simulink model "Control_Scheme_Cartesian_PID_Simulink"  (R2021a)
settings: Solver=VariableStepAuto  StartTime=0.0  StopTime=8  RelTol=1e-20
libraries: simulink x10, pid_lib x6
(part 1 of 2)
settings Model: Creator=WU  LastModifiedBy=WU

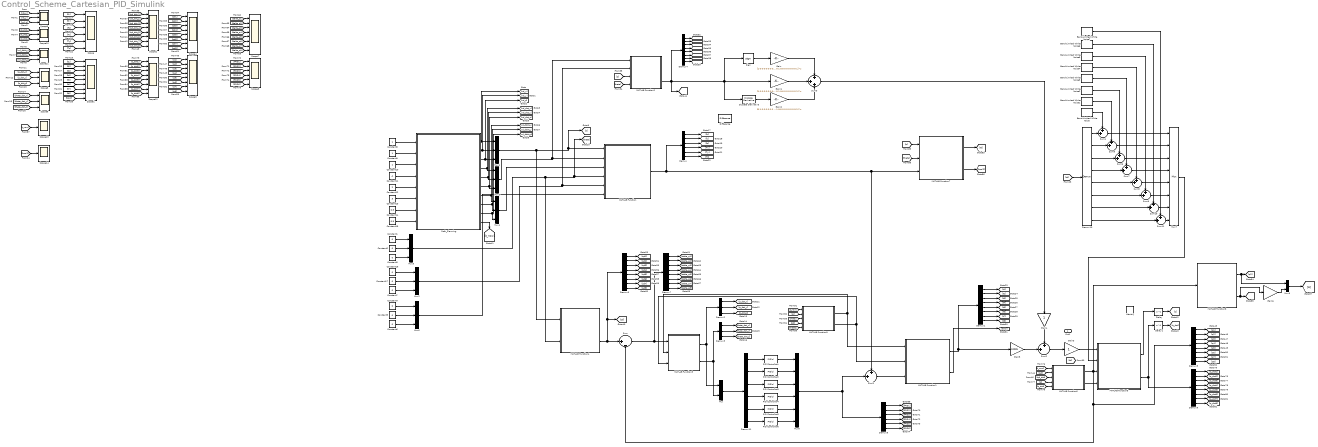
== system Control_Scheme_Cartesian_PID_Simulink ==
  Band-Limited White Noise : simulink/Sources/Band-Limited White Noise  Cov=[50]  Ts=0.001  seed=[23348]
  Band-Limited White Noise1 : simulink/Sources/Band-Limited White Noise  Cov=[50]  Ts=0.001  seed=[23347]
  Band-Limited White Noise2 : simulink/Sources/Band-Limited White Noise  Cov=[50]  Ts=0.001  seed=[23346]
  Band-Limited White Noise3 : simulink/Sources/Band-Limited White Noise  Cov=[50]  Ts=0.001  seed=[23345]
  Band-Limited White Noise4 : simulink/Sources/Band-Limited White Noise  Cov=[50]  Ts=0.001  seed=[23344]
  Band-Limited White Noise5 : simulink/Sources/Band-Limited White Noise  Cov=[50]  Ts=0.001  seed=[23343]
  Band-Limited White Noise6 : simulink/Sources/Band-Limited White Noise  Cov=[50]  Ts=0.001  seed=[23342]
  Band-Limited White Noise7 : simulink/Sources/Band-Limited White Noise  Cov=[50]  Ts=0.001  seed=[23341]
  Constant1 : Constant  Value=0  VectorParams1D=off
  Constant10 : Constant
  Constant11 : Constant  Value=-1
  Constant12 : Constant  Value=2
  Constant13 : Constant  Value=3
  Constant14 : Constant  Value=0.5
  Constant15 : Constant  Value=0.5
  Constant16 : Constant  Value=0  VectorParams1D=off
  Constant{2..3,5..7,17} (6 alike) : Constant  Value=0
  Constant4 : Constant  Value=0  VectorParams1D=off
  Constant8 : Constant  VectorParams1D=off
  Constant9 : Constant
  Delay : Delay  DelayLength=1
  Delay1 : Delay  DelayLength=1
  Demux : Demux  Outputs=6
      settings: DisplayOption=none
  Demux{1,4..7,9..10} (7 alike) : Demux  Outputs=8
      Demux1 settings: DisplayOption=none
      Demux10 settings: DisplayOption=none
      Demux4 settings: DisplayOption=none
  Demux11 : Demux  Outputs=6
      settings: DisplayOption=none
  Demux2 : Demux  Outputs=3
      settings: DisplayOption=none
  Demux3 : Demux  Outputs=3
      settings: DisplayOption=none
  Demux8 : Demux  Outputs=6
      settings: DisplayOption=none
  Difference : simulink/Discrete/Difference  ICPrevInput=0.0  OutMin=[]  OutMax=[]  OutDataType=fixdt(1, 16)  OutScaling=2^-10  DoSatur=off
  Discrete Derivative : simulink/Discrete/Discrete Derivative  gainval=1.0  ICPrevScaledInput=0.0  OutMin=[]  OutMax=[]  OutDataType=fixdt(1, 16)  OutScaling=2^-10  DoSatur=off
  Gain : Gain  Gain=[1 0 0 0 0 0 0 0;0 1 0 0 0 0 0 0;0 0 1 0 0 0 0 0;0 0 0 1 0 0 0 0;0 0 0 0 1 0 0 0;0 0 0 0 0 1 0 0;0 0 0 0 0 0 1 0;0 0 0 0 0 0 0 1]  Multiplication=Matrix(K*u) (u vector)
  Gain1 : Gain  Gain=[1 0 0 0 0 0 0 0;0 1 0 0 0 0 0 0;0 0 1 0 0 0 0 0;0 0 0 1 0 0 0 0;0 0 0 0 1 0 0 0;0 0 0 0 0 1 0 0;0 0 0 0 0 0 1 0;0 0 0 0 0 0 0 1]  Multiplication=Matrix(K*u) (u vector)
  Gain2 : Gain  Gain=[0.1 0 0 0 0 0 0 0;0 0.1 0 0 0 0 0 0;0 0 0.1 0 0 0 0 0;0 0 0 0.1 0 0 0 0;0 0 0 0 0.1 0 0 0;0 0 0 0 0 0.1 0 0;0 0 0 0 0 0 0.1 0;0 0 0 0 0 0 0 0.1]  Multiplication=Matrix(K*u) (u vector)
  Gain3 : Gain
  Gain4 : Gain
  Gain5 : Gain  Gain=0.0225
  Gain6 : Gain  Gain=3.14/180
  MATLAB Function : MATLAB Function  TreatAsAtomicUnit=on
  MATLAB Function1 : MATLAB Function  TreatAsAtomicUnit=on
  MATLAB Function2 : MATLAB Function  TreatAsAtomicUnit=on
  MATLAB Function3 : MATLAB Function  TreatAsAtomicUnit=on
  MATLAB Function4 : MATLAB Function  TreatAsAtomicUnit=on
  MATLAB Function5 : MATLAB Function  TreatAsAtomicUnit=on
  MATLAB Function6 : MATLAB Function  TreatAsAtomicUnit=on
  MATLAB Function7 : MATLAB Function  TreatAsAtomicUnit=on
  MATLAB Function8 : MATLAB Function  TreatAsAtomicUnit=on
  MATLAB Function9 : MATLAB Function  TreatAsAtomicUnit=on
  Memory : Memory
  Mux : Mux  Inputs=2
  Mux{1..6} (6 alike) : Mux  Inputs=3
  Mux7 : Mux  Inputs=8
  Mux8 : Mux  Inputs=6
  Mux9 : Mux  Inputs=2
  PID Controller{1..6} (6 alike) : pid_lib/PID Controller  Controller=PID  Form=Parallel  TimeDomain=Discrete-time  UseExternalTs=off  SampleTime=-1  IntegratorMethod=Forward Euler  FilterMethod=Forward Euler  ControllerParametersSource=internal  P=-150000  I=-1000  D=-100  UseFilter=on  N=100  TunerSelectOption=Transfer Function Based (PID Tuner App)  InitialConditionSource=internal  InitialConditionForIntegrator=0  InitialConditionForFilter=0  DifferentiatorICPrevScaledInput=0  ExternalReset=none  TrackingMode=off  Kt=1  LimitOutput=off  SatLimitsSource=internal  UpperSaturationLimit=inf  LowerSaturationLimit=-inf  LinearizeAsGain=on  AntiWindupMode=none  Kb=1  POutMin=[]  POutMax=[]  IOutMin=[]  IOutMax=[]  DOutMin=[]  DOutMax=[]  NOutMin=[]  NOutMax=[]  SumOutMin=[]  SumOutMax=[]  SaturationOutMin=[]  SaturationOutMax=[]  PParamMin=[]  PParamMax=[]  IParamMin=[]  IParamMax=[]  DParamMin=[]  DParamMax=[]  NParamMin=[]  NParamMax=[]  KbParamMin=[]  KbParamMax=[]  KtParamMin=[]  KtParamMax=[]  KbOutMin=[]  KbOutMax=[]  KtOutMin=[]  KtOutMax=[]  IntegratorOutMin=[]  IntegratorOutMax=[]  FilterOutMin=[]  FilterOutMax=[]  SumI1OutMin=[]  SumI1OutMax=[]  SumI2OutMin=[]  SumI2OutMax=[]  SumI3OutMin=[]  SumI3OutMax=[]  SumI4OutMin=[]  SumI4OutMax=[]  SumDOutMin=[]  SumDOutMax=[]  DifferentiatorOutMin=[]  DifferentiatorOutMax=[]  FilterDiffOutCoefMin=[]  FilterDiffOutCoefMax=[]  ReciprocalOutMin=[]  ReciprocalOutMax=[]  SumDenOutMin=[]  SumDenOutMax=[]  SumNumOutMin=[]  SumNumOutMax=[]  DivideOutMin=[]  DivideOutMax=[]  UdiffTsProdOutMin=[]  UdiffTsProdOutMax=[]  NTsProdOutMin=[]  NTsProdOutMax=[]  UintegralTsProdOutMin=[]  UintegralTsProdOutMax=[]  UngainTsProdOutMin=[]  UngainTsProdOutMax=[]  IntegratorContinuousStateAttributes=''  IntegratorStateMustResolveToSignalObject=off  IntegratorRTWStateStorageClass=Auto  FilterContinuousStateAttributes=''  FilterStateMustResolveToSignalObject=off  FilterRTWStateStorageClass=Auto  ParallelPVariant=InternalParameters  IdealPVariant=Disabled  IVariant=InternalParameters  DVariant=InternalParameters  IntegratorVariant=Discrete  SatVariant=Disabled  AWVariant=Passthrough  PCopyVariant=Disabled  TRVariant=Disabled  FdbkBlocksVariant=Forward  IdealPFdbkVariant=Disabled  SatFdbkVariant=Disabled  DerivativeFilterVariant=ForwardEulerFilter  NVariant=InternalParameters  NCopyVariant=Disabled  FilterICVariant=InternalICsFilter  IntegratorICVariant=InternalICs  ExternalResetVariant=Disabled  TRSumVariant=Passthrough  SumFdbkVariant=Disabled  SumVariant=Sum_PID  TsampFilterVariant=InternalTs  TsampNgainVariant=Passthrough  TsampIntegralVariant=Passthrough  ExternalSaturationOutDataTypeStr=Inherit: Same as second input
  Path_Planning : Subsystem
  Scope : Scope  NumInputPorts=6
  Scope1 : Scope  NumInputPorts=9
  Scope{5..6,9..11} (5 alike) : Scope  NumInputPorts=3
  Scope{2..4,7,12} (5 alike) : Scope  NumInputPorts=8
  Scope13 : Scope
  Scope14 : Scope
  Scope8 : Scope  NumInputPorts=6
  Sign : Signum
  Sum : Sum  Inputs=|+-
  Sum{1..2,4..11} (10 alike) : Sum  Inputs=++|
  Sum3 : Sum  Inputs=+++
  Out1 : Outport
  wires:
  Constant8/1 -> Path_Planning/1(xinit_x)  "xinit_x"
  Constant9/1 -> Path_Planning/2(xinit_y)  "xinit_y"
  Constant10/1 -> Path_Planning/3(xinit_z)  "xinit_z"
  Constant11/1 -> Path_Planning/4(xend_x)  "xend_x"
  Constant12/1 -> Path_Planning/5(xend_y)  "xend_y"
  Constant13/1 -> Path_Planning/6(xend_z)  "xend_z"
  Constant14/1 -> Path_Planning/7(vm)  "vm"
  Constant15/1 -> Path_Planning/8(am)  "am"
  Constant7/1 -> Mux2/3  "theta_dot_z"
  Constant17/1 -> Mux2/2  "theta_dot_y"
  Constant16/1 -> Mux2/1  "theta_dot_x"
  MATLAB Function/1(f) -> MATLAB Function7/3(we), Sum1/1, Demux/1  "fFF"
  Demux/1 -> [fx]  "fx"
  Demux/3 -> [fz]  "fz"
  Demux/4 -> [Tx]  "Tx"
  Demux/5 -> [Ty]  "Ty"
  Demux/6 -> [Tz]  "Tz"
  Path_Planning/1(xd_x) -> [xd_x], Mux1/1
  Path_Planning/3(xd_z) -> [xd_z], Mux1/3
  Path_Planning/4(xd_dot_x) -> [xd_dot_x], Mux3/1
  Path_Planning/5(xd_dot_y) -> [xd_dot_y], Mux3/2
  Path_Planning/6(xd_dot_z) -> [xd_dot_z], Mux3/3
  Path_Planning/7(xd_ddot_x) -> [xd_ddot_x], Mux4/1
  Path_Planning/8(xd_ddot_y) -> [xd_ddot_y], Mux4/2
  Path_Planning/9(xd_ddot_z) -> [xd_ddot_z], Mux4/3
  Path_Planning/2(xd_y) -> [xd_y], Mux1/2
  Constant1/1 -> Mux5/1  "theta_x"
  Constant2/1 -> Mux5/2  "theta_y"
  Constant3/1 -> Mux5/3  "theta_z"
  Mux5/1 -> MATLAB Function4/2(theta), [theta], MATLAB Function/4(theta)  "theta"
  MATLAB Function1/1(t) -> Gain5/1, Demux1/1  "t"
  Demux1/1 -> [t1]  "t1"
  Demux1/2 -> [t2]  "t2"
  Demux1/3 -> [t3]  "t3"
  Demux1/4 -> [t4]  "t4"
  Demux1/5 -> [t5]  "t5"
  Demux1/6 -> [t6]  "t6"
  Demux1/7 -> [t7]  "t7"
  Demux1/8 -> [t8]  "t8"
  MATLAB Function1/2(bool) -> [bool]
  MATLAB Function3/1(p_dot) -> Mux/1, Demux2/1
  Demux2/1 -> [p_dot_x]
  Demux2/2 -> [p_dot_y]
  Demux2/3 -> [p_dot_z]
  Demux3/1 -> [theta_dot_x]
  Demux3/3 -> [theta_dot_z]
  Demux3/2 -> [theta_dot_y]
  MATLAB Function3/2(theta_dot) -> Demux3/1, Mux/2
  Mux1/1 -> [p], MATLAB Function/1(p), MATLAB Function4/1(p)  "p"
  Mux3/1 -> MATLAB Function/2(p_dot), MATLAB Function2/1(p_dot)  "p_dot"
  Mux4/1 -> MATLAB Function/3(p_ddot)  "p_ddot"
  Constant6/1 -> Mux6/3  "theta_ddot_z"
  Constant4/1 -> Mux6/1  "theta_ddot_x"
  Constant5/1 -> Mux6/2  "theta_ddot_y"
  Mux2/1 -> MATLAB Function2/2(theta_dot), MATLAB Function/5(theta_dot)  "theta_dot"
  Mux6/1 -> MATLAB Function/6(theta_ddot)  "theta_ddot"
  MATLAB Function4/2(q) -> Demux6/1, [qd], Sum/1  "qd"
  [xd_x] -> Scope9/1
  [xd_y] -> Scope9/2
  [xd_z] -> Scope9/3
  [xd_dot_x] -> Scope10/1
  [xd_dot_y] -> Scope10/2
  [xd_ddot_x] -> Scope11/1
  [xd_ddot_y] -> Scope11/2
  [xd_ddot_z] -> Scope11/3
  Sum/1 -> Demux7/1, MATLAB Function3/1(q_dot)  "delta_q"
  MATLAB Function9/1(p_out) -> MATLAB Function3/2(p), MATLAB Function1/1(p)
  [p_dot_x] -> Scope5/1
  [p_dot_y] -> Scope5/2
  [p_dot_z] -> Scope5/3
  [theta_dot_x] -> Scope6/1
  [theta_dot_y] -> Scope6/2
  [theta_dot_z] -> Scope6/3
  Demux/2 -> [fy]  "fy"
  [fx] -> Scope/1
  [fy] -> Scope/2
  [fz] -> Scope/3
  [Tx] -> Scope/4
  [Ty] -> Scope/5
  [Tz] -> Scope/6
  MATLAB Function9/2(theta_out) -> MATLAB Function3/3(theta), MATLAB Function1/2(theta)
  [t1] -> Scope1/1
  [t4] -> Scope1/4
  [t8] -> Scope1/8
  [t5] -> Scope1/5
  [bool] -> Scope1/9
  [t7] -> Scope1/7
  [t6] -> Scope1/6
  [t3] -> Scope1/3
  [t2] -> Scope1/2
  [xd_dot_z] -> Scope10/3
  [p] -> MATLAB Function2/3(p)
  [theta] -> MATLAB Function2/4(theta)
  MATLAB Function2/2(q_dot) -> [qd_dot], Discrete Derivative/1, Gain1/1, Sign/1, Demux4/1  "q_dot"
  Demux4/1 -> [qd_dot_1]
  Demux4/2 -> [qd_dot_2]
  Demux4/3 -> [qd_dot_3]
  Demux4/4 -> [qd_dot_4]
  Demux4/5 -> [qd_dot_5]
  Demux4/6 -> [qd_dot_6]
  Demux4/7 -> [qd_dot_7]
  Demux4/8 -> [qd_dot_8]
  [qd_dot_1] -> Scope2/1
  [qd_dot_2] -> Scope2/2
  [qd_dot_4] -> Scope2/4
  [qd_dot_5] -> Scope2/5
  [qd_dot_6] -> Scope2/6
  [qd_dot_7] -> Scope2/7
  [qd_dot_8] -> Scope2/8
  [qd_dot_3] -> Scope2/3
  Discrete Derivative/1 -> Gain2/1
  Sign/1 -> Gain/1
  Gain1/1 -> Sum3/2
  Gain/1 -> Sum3/1
  Gain2/1 -> Sum3/3
  Gain3/1 -> MATLAB Function5/1(tao_in)  "tao_in"
  MATLAB Function5/1(q) -> Delay/1  "q"
  Path_Planning/10(t_now) -> [t_now]
  Demux5/1 -> [q1]
  Demux5/2 -> [q2]
  Demux5/3 -> [q3]
  Demux5/4 -> [q4]
  Demux5/7 -> [q7]
  Demux5/6 -> [q6]
  Demux5/8 -> [q8]
  Demux5/5 -> [q5]
  Demux6/3 -> [qd3]
  Demux6/4 -> [qd4]
  Demux6/7 -> [qd7]
  Demux6/1 -> [qd1]
  Demux6/5 -> [qd5]
  Demux6/6 -> [qd6]
  Demux6/8 -> [qd8]
  Demux6/2 -> [qd2]
  [q5] -> Scope3/5
  [q4] -> Scope3/4
  [q7] -> Scope3/7
  [q8] -> Scope3/8
  [q6] -> Scope3/6
  [q1] -> Scope3/1
  [q3] -> Scope3/3
  [q2] -> Scope3/2
  [qd8] -> Scope4/8
  [qd7] -> Scope4/7
  [qd5] -> Scope4/5
  [qd6] -> Scope4/6
  [qd2] -> Scope4/2
  [qd4] -> Scope4/4
  [qd3] -> Scope4/3
  [qd1] -> Scope4/1
  Demux7/8 -> [delta_q8]
  Demux7/2 -> [delta_q2]
  Demux7/3 -> [delta_q3]
  Demux7/7 -> [delta_q7]
  Demux7/4 -> [delta_q4]
  Demux7/5 -> [delta_q5]
  Demux7/1 -> [delta_q1]
  Demux7/6 -> [delta_q6]
  [delta_q1] -> Scope7/1
  [delta_q8] -> Scope7/8
  [delta_q3] -> Scope7/3
  [delta_q4] -> Scope7/4
  [delta_q5] -> Scope7/5
  [delta_q7] -> Scope7/7
  [delta_q6] -> Scope7/6
  [delta_q2] -> Scope7/2
  Demux8/4 -> [fPID4]  "fPID4"
  Demux8/5 -> [fPID5]  "fPID5"
  Demux8/1 -> [fPID1]  "fPID1"
  Demux8/2 -> [fPID2]  "fPID2"
  Demux8/3 -> [fPID3]  "fPID3"
  Demux8/6 -> [fPID6]  "fPID6"
  [fPID4] -> Scope8/4
  [fPID3] -> Scope8/3
  [fPID1] -> Scope8/1
  [fPID6] -> Scope8/6
  [fPID2] -> Scope8/2
  [fPID5] -> Scope8/5
  [qd] -> MATLAB Function6/2(qd)
  [t_now] -> MATLAB Function6/1(t)
  [qd_dot] -> MATLAB Function6/3(qd_dot)
  [q] -> MATLAB Function6/4(q)
  [q_dot] -> MATLAB Function6/5(q_dot)
  MATLAB Function6/1(q_1) -> Demux5/1, Sum/2, MATLAB Function8/1(q), MATLAB Function5/3(q_1)  "q"
  Delay/1 -> [q]
  MATLAB Function5/2(q_dot) -> Delay1/1, Demux9/1  "q_dot"
  Demux9/3 -> [q_dot3]
  Demux9/2 -> [q_dot2]
  Demux9/1 -> [q_dot1]
  Demux9/7 -> [q_dot7]
  Demux9/5 -> [q_dot5]
  Demux9/4 -> [q_dot4]
  Demux9/8 -> [q_dot8]
  Demux9/6 -> [q_dot6]
  [q_dot2] -> Scope12/2
  [q_dot8] -> Scope12/8
  [q_dot6] -> Scope12/6
  [q_dot7] -> Scope12/7
  [q_dot5] -> Scope12/5
  [q_dot3] -> Scope12/3
  [q_dot1] -> Scope12/1
  [q_dot4] -> Scope12/4
  [t_now] -> Scope13/1
  [theta] -> MATLAB Function7/2(theta)
  [p] -> MATLAB Function7/1(p)
  MATLAB Function7/1(t) -> [td]  "tTD"
  Sum2/1 -> Gain3/1
  Gain5/1 -> Sum2/2  "tao"
  MATLAB Function6/2(q_dot_1) -> MATLAB Function5/4(q_dot_1)  "q_dot_1"
  MATLAB Function8/1(p) -> Mux9/1, [p2]
  MATLAB Function8/2(theta) -> Gain6/1, [theta2]
  [p2] -> MATLAB Function9/4(p2)
  [t_now] -> MATLAB Function9/1(t_now)
  [theta2] -> MATLAB Function9/5(theta2)
  [theta] -> MATLAB Function9/3(theta)
  [p] -> MATLAB Function9/2(p)
  Gain4/1 -> Sum2/1  "taoff"
  Sum3/1 -> Gain4/1  "tFF"
  MATLAB Function7/2(bool) -> [bool2]
  [td] -> Demux10/1
  Demux10/1 -> Sum4/2
  Band-Limited White Noise/1 -> Sum4/1
  Sum4/1 -> Mux7/1
  Demux10/2 -> Sum5/2
  Sum5/1 -> Mux7/2
  Demux10/3 -> Sum6/2
  Sum6/1 -> Mux7/3
  Demux10/4 -> Sum7/2
  Sum7/1 -> Mux7/4
  Demux10/5 -> Sum8/2
  Sum8/1 -> Mux7/5
  Demux10/6 -> Sum9/2
  Sum9/1 -> Mux7/6
  Demux10/7 -> Sum10/2
  Sum10/1 -> Mux7/7
  Demux10/8 -> Sum11/2
  Sum11/1 -> Mux7/8
  Band-Limited White Noise1/1 -> Sum5/1
  Band-Limited White Noise2/1 -> Sum6/1
  Band-Limited White Noise3/1 -> Sum7/1
  Band-Limited White Noise4/1 -> Sum8/1
  Band-Limited White Noise5/1 -> Sum9/1
  Band-Limited White Noise6/1 -> Sum10/1
  Band-Limited White Noise7/1 -> Sum11/1
  Mux/1 -> Demux11/1  "delta_x"
  Demux11/1 -> PID Controller1/1
  Demux11/2 -> PID Controller2/1
  PID Controller1/1 -> Mux8/1  "fPID"
  PID Controller2/1 -> Mux8/2  "fPID"
  Demux11/4 -> PID Controller4/1
  PID Controller4/1 -> Mux8/4  "fPID"
  Demux11/3 -> PID Controller3/1
  PID Controller3/1 -> Mux8/3  "fPID"
  PID Controller5/1 -> Mux8/5  "fPID"
  PID Controller6/1 -> Mux8/6  "fPID"
  Demux11/6 -> PID Controller6/1
  Mux8/1 -> Sum1/2, Demux8/1  "fPID"
  [bool2] -> Scope14/1
  Delay1/1 -> [q_dot]
  Mux7/1 -> MATLAB Function5/2(t_in)
  Mux9/1 -> [A]  "x"
  Gain6/1 -> Mux9/2
  Demux11/5 -> PID Controller5/1
  Sum1/1 -> MATLAB Function1/3(we)  "f"

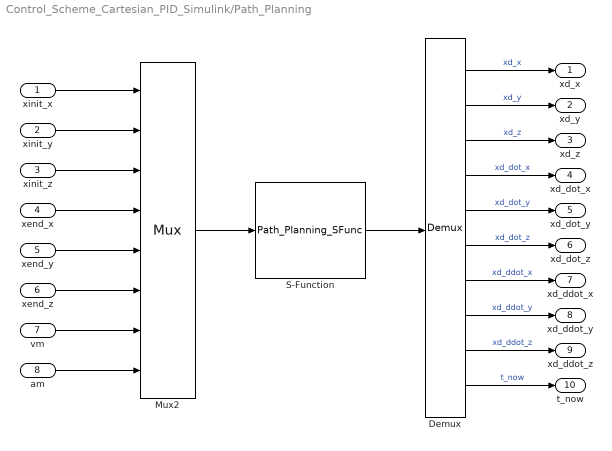
== system Control_Scheme_Cartesian_PID_Simulink/Path_Planning ==
  xinit_x : Inport
  xinit_y : Inport  Port=2
  xinit_z : Inport  Port=3
  xend_x : Inport  Port=4
  xend_y : Inport  Port=5
  xend_z : Inport  Port=6
  vm : Inport  Port=7
  am : Inport  Port=8
  Demux : Demux  Outputs=10
      settings: DisplayOption=none
  Mux2 : Mux  Inputs=8
  S-Function : S-Function  FunctionName=Path_Planning_SFunc  SFunctionDeploymentMode=off  EnableBusSupport=off
  xd_x : Outport
  xd_y : Outport  Port=2
  xd_z : Outport  Port=3
  xd_dot_x : Outport  Port=4
  xd_dot_y : Outport  Port=5
  xd_dot_z : Outport  Port=6
  xd_ddot_x : Outport  Port=7
  xd_ddot_y : Outport  Port=8
  xd_ddot_z : Outport  Port=9
  t_now : Outport  Port=10
  wires:
  Demux/7 -> xd_ddot_x/1  "xd_ddot_x"
  vm/1 -> Mux2/7
  xinit_y/1 -> Mux2/2
  Demux/1 -> xd_x/1  "xd_x"
  Demux/4 -> xd_dot_x/1  "xd_dot_x"
  Demux/5 -> xd_dot_y/1  "xd_dot_y"
  Demux/9 -> xd_ddot_z/1  "xd_ddot_z"
  Demux/8 -> xd_ddot_y/1  "xd_ddot_y"
  Demux/3 -> xd_z/1  "xd_z"
  Demux/6 -> xd_dot_z/1  "xd_dot_z"
  Demux/2 -> xd_y/1  "xd_y"
  xend_y/1 -> Mux2/5
  Mux2/1 -> S-Function/1
  S-Function/1 -> Demux/1
  xend_z/1 -> Mux2/6
  xend_x/1 -> Mux2/4
  xinit_z/1 -> Mux2/3
  xinit_x/1 -> Mux2/1
  am/1 -> Mux2/8
  Demux/10 -> t_now/1  "t_now"

== matlab function Control_Scheme_Cartesian_PID_Simulink/MATLAB Function9 ==
  data: t_now input; p_out output; p input; theta input; p2 input; theta2 input; theta_out output
function [p_out,theta_out]= Select_p_and_theta(t_now,p,theta,p2,theta2)
p_out=zeros(3,1);
theta_out=zeros(3,1);

if t_now<=1e-3
    p_out=p;
    theta_out=theta;
else
    p_out=p2;
    theta_out=theta2;
end
p_out=p;
theta_out=theta;


end

== matlab function Control_Scheme_Cartesian_PID_Simulink/MATLAB Function1 ==
  data: p input; t output; theta input; we input; bool output
function [t,bool] = Tension_Distribution_Func(p,theta,we)
% 求解索力分布的函数
% 输入：p 动平台位置 3*1
%      theta 动平台坐标系XYZ欧拉角 3*1
%      we 动平台受到的wrench 6*1(包含本身质量)
% 输出：t 绳索的张力的大小 8*1

g=9.81; %重力加速度
theta=theta';
x=theta(1);
y=theta(2);
z=theta(3);
Rxyz=Theta2RotationMatrix_Func(x,y,z);
f=we;
%% CoGiRo的参数 8绳索6自由度的CDPRs
% ai的定义
a1=[-7.5 -5.5 6]';
a2=[-7.5 -5.5 6]';
a3=[-7.5 5.5 6]';
a4=[-7.5 5.5 6]';
a5=[7.5 5.5 6]';
a6=[7.5 5.5 6]';
a7=[7.5 -5.5 6]';
a8=[7.5 -5.5 6]';
% bi的定义
b1=Rxyz*[0.5 -0.5 0]';
b2=Rxyz*[-0.5 0.5 1]';
b3=Rxyz*[-0.5 -0.5 0]';
b4=Rxyz*[0.5 0.5 1]';
b5=Rxyz*[-0.5 0.5 0]';
b6=Rxyz*[0.5 -0.5 1]';
b7=Rxyz*[0.5 0.5 0]';
b8=Rxyz*[-0.5 -0.5 1]';
% 绳索张力的上下限
tM=1000;
tm=10;
%% li=ai-bi-p,然后归一化li得到si=li/norm(li)
% li=ai-bi-p
l1=a1-b1-p;
l2=a2-b2-p;
l3=a3-b3-p;
l4=a4-b4-p;
l5=a5-b5-p;
l6=a6-b6-p;
l7=a7-b7-p;
l8=a8-b8-p;
% for i=1:8
%     expr=['l',num2str(i),'=a',num2str(i),'-b',num2str(i),'-p;'];
%     eval(expr);
% end
% si=li/norm(li)
s1=l1/norm(l1);
s2=l2/norm(l2);
s3=l3/norm(l3);
s4=l4/norm(l4);
s5=l5/norm(l5);
s6=l6/norm(l6);
s7=l7/norm(l7);
s8=l8/norm(l8);

% for i=1:8
%     expr=['s',num2str(i),'=l',num2str(i),'./norm(l',num2str(i),');'];
%     eval(expr);
% end

%% 构建W矩阵
% wi=[si;cross(bi,si)]
w1=[s1;cross(b1,s1)];
w2=[s2;cross(b2,s2)];
w3=[s3;cross(b3,s3)];
w4=[s4;cross(b4,s4)];
w5=[s5;cross(b5,s5)];
w6=[s6;cross(b6,s6)];
w7=[s7;cross(b7,s7)];
w8=[s8;cross(b8,s8)];
W=[w1 w2 w3 w4 w5 w6 w7 w8];

W_plus=pinv(W);
N=null(W);
tp=W_plus*f;

tm_vec=[tm;tm;tm;tm;tm;tm;tm;tm;];
tM_vec=[tM;tM;tM;tM;tM;tM;tM;tM;];

% line_select=[];
% langda_select=[];

find=0;
k_vector_all=[1;2;3;4;5;6;7;8];

%% 寻找第一个顶点vinit
i=1;
j=2;
bi=tm;
bj=tm;
bk_1=0;
bk_2=0;
ni=N(i,:);
nj=N(j,:);
tpi=tp(i,:);
tpj=tp(j,:);
A=[ni;nj];
b=[bi-tpi;bj-tpj];
langda=A\b; %2*1向量
vij=langda;

% line_select=[line_select;j];
% line_select=[line_select;i];
line_select=[i];

lk_1=i;
lk_2=j;

% line_find=[];
% line_find=[line_find;1];
% line_find=[line_find;2];
line_find=[i;j];

for i=3:8
    ni_2=N(i,:);
    tpi_2=tp(i,:);
    if ni_2*langda>=tm-tpi_2 & ni_2*langda<=tM-tpi_2
        line_find=[line_find;i];
    end
    
end

langda_select=[vij];


k_vector=setdiff(k_vector_all,line_select);

%% 循环找下一个节点，直到找到vk==vf
vk=[1e30;1e30];
% alpah_v=[1e30;1e30];
alpah_v=[1e30];
vk_1=vij;
nk_1=ni;
nk_2=nj;
nk_1_vertical=null(nk_1)';
nk_2_vertical=null(nk_2)';
l=0;
bk=0;
tpk=0;
count=0;
find2=0;
vf=vij;
vf_count=count+1;
nk_1_vertical_final=[0 0];
while(1)
%     alpah_k=[1e30;1e30];
    alpah_k=[1e30];
    count=count+1;
    find2=0;
    nk_1_vertical_final=[0 0];
    for i=1:length(k_vector)
        k=k_vector(i);
        nk=N(k,:);
        tpk=tp(k,:);
        
        % 考虑bj=tm情况
        if bk_2==0           
            nk_1_vertical_1=[nk_1(2) -nk_1(1)];
            nk_1_vertical_2=[-nk_1(2) nk_1(1)];
%             nk_1_vertical_1=[-nk_1(2) nk_1(1)];
%             nk_1_vertical_2=[nk_1(2) -nk_1(1)];
            if nk_2*nk_1_vertical_1'>=0
                nk_1_vertical=nk_1_vertical_1;
            else
                nk_1_vertical=nk_1_vertical_2;
            end           
            
            if nk*nk_1_vertical'>0
                if k==lk_2
                    if nk*vk_1<=tm-tpk
                        alpah_k=(tM-tpk-nk*vk_1)/(nk*nk_1_vertical');
                        bk_tmp=1;
                    elseif nk*vk_1>tm-tpk & nk*vk_1<=tM-tpk
                        alpah_k=(tM-tpk-nk*vk_1)/(nk*nk_1_vertical');
                        bk_tmp=1;
                    else
                        bk_tmp=0;
                    end
%                     if nk*vk_1>tm-tpk & nk*vk_1<=tM-tpk
%                         alpah_k=(tM-tpk-nk*vk_1)/(nk*nk_1_vertical');
%                         bk_tmp=1;
%                     end
                else
                    if nk*vk_1<=tm-tpk
                        alpah_k=(tm-tpk-nk*vk_1)/(nk*nk_1_vertical');
                        bk_tmp=0;
                    elseif nk*vk_1>tm-tpk & nk*vk_1<=tM-tpk
                        alpah_k=(tM-tpk-nk*vk_1)/(nk*nk_1_vertical');
                        bk_tmp=1;
                    else
                        bk_tmp=0;
                    end
%                     if nk*vk_1>tm-tpk & nk*vk_1<=tM-tpk
%                         alpah_k=(tM-tpk-nk*vk_1)/(nk*nk_1_vertical');
%                         bk_tmp=1;
%                     end
                end
                if (alpah_k<alpah_v) & alpah_k>=1e-6
                    alpah_v=alpah_k;
                    l=k;
                    find2=1;
                    nk_1_vertical_final=nk_1_vertical;
                    bk=bk_tmp;
                else
                    
                end
            end

            if nk*nk_1_vertical'<0
                if k==lk_2
                    if nk*vk_1>=tM-tpk
                        alpah_k=(tm-tpk-nk*vk_1)/(nk*nk_1_vertical');
                        bk_tmp=0;
                    elseif nk*vk_1>=tm-tpk & nk*vk_1<tM-tpk
                        alpah_k=(tm-tpk-nk*vk_1)/(nk*nk_1_vertical');
                        bk_tmp=0;
                    else
                        bk_tmp=0;
                    end
%                     if nk*vk_1>=tm-tpk & nk*vk_1<tM-tpk
%                         alpah_k=(tm-tpk-nk*vk_1)/(nk*nk_1_vertical');
%                         bk_tmp=0;
%                     end
                else
                    if nk*vk_1>=tM-tpk
                        alpah_k=(tM-tpk-nk*vk_1)/(nk*nk_1_vertical');
                        bk_tmp=1;
                    elseif nk*vk_1>=tm-tpk & nk*vk_1<tM-tpk
                        alpah_k=(tm-tpk-nk*vk_1)/(nk*nk_1_vertical');
                        bk_tmp=0;
                    else
                        bk_tmp=0;
                    end
%                     if nk*vk_1>=tm-tpk & nk*vk_1<tM-tpk
%                         alpah_k=(tm-tpk-nk*vk_1)/(nk*nk_1_vertical');
%                         bk_tmp=0;
%                     end
                end
                if (alpah_k<alpah_v) & alpah_k>=1e-6
                    alpah_v=alpah_k;
                    l=k;
                    find2=1;
                    nk_1_vertical_final=nk_1_vertical;
                    bk=bk_tmp;
                else
                    
                end
            end
        
        % 考虑bk=tM的情况
        elseif bk_2==1
            nk_1_vertical_1=[nk_1(2) -nk_1(1)];
            nk_1_vertical_2=[-nk_1(2) nk_1(1)];
%             nk_1_vertical_1=[-nk_1(2) nk_1(1)];
%             nk_1_vertical_2=[nk_1(2) -nk_1(1)];
            if nk_2*nk_1_vertical_1'<=0
                nk_1_vertical=nk_1_vertical_1;
            else
                nk_1_vertical=nk_1_vertical_2;
            end

            if nk*nk_1_vertical'>0
                if k==lk_2
                    if nk*vk_1<=tm-tpk
                        alpah_k=(tM-tpk-nk*vk_1)/(nk*nk_1_vertical');
                        bk_tmp=1;
                    elseif nk*vk_1>tm-tpk & nk*vk_1<=tM-tpk
                        alpah_k=(tM-tpk-nk*vk_1)/(nk*nk_1_vertical');
                        bk_tmp=1;
                    else
                        bk_tmp=0;
                    end
%                     if nk*vk_1>tm-tpk & nk*vk_1<=tM-tpk
%                         alpah_k=(tM-tpk-nk*vk_1)/(nk*nk_1_vertical');
%                         bk_tmp=1;
%                     end
                else
                    if nk*vk_1<=tm-tpk
                        alpah_k=(tm-tpk-nk*vk_1)/(nk*nk_1_vertical');
                        bk_tmp=0;
                    elseif nk*vk_1>tm-tpk & nk*vk_1<=tM-tpk
                        alpah_k=(tM-tpk-nk*vk_1)/(nk*nk_1_vertical');
                        bk_tmp=1;
                    else
                        bk_tmp=0;
                    end
%                     if nk*vk_1>tm-tpk & nk*vk_1<=tM-tpk
%                         alpah_k=(tM-tpk-nk*vk_1)/(nk*nk_1_vertical');
%                         bk_tmp=1;
%                     end
                end
                if (alpah_k<alpah_v) & alpah_k>=1e-6
                    alpah_v=alpah_k;
                    l=k;
                    find2=1;
                    nk_1_vertical_final=nk_1_vertical;
                    bk=bk_tmp;
                else
                    
                end
            end

            if nk*nk_1_vertical'<0
                if k==lk_2
                    if nk*vk_1>=tM-tpk
                        alpah_k=(tm-tpk-nk*vk_1)/(nk*nk_1_vertical');
                        bk_tmp=0;
                    elseif nk*vk_1>=tm-tpk & nk*vk_1<tM-tpk
                        alpah_k=(tm-tpk-nk*vk_1)/(nk*nk_1_vertical');
                        bk_tmp=0;
                    else
                        bk_tmp=0;
                    end
%                     if nk*vk_1>=tm-tpk & nk*vk_1<tM-tpk
%                         alpah_k=(tm-tpk-nk*vk_1)/(nk*nk_1_vertical');
%                         bk_tmp=0;
%                     end
                else
                    if nk*vk_1>=tM-tpk
                        alpah_k=(tM-tpk-nk*vk_1)/(nk*nk_1_vertical');
                        bk_tmp=1;
                    elseif nk*vk_1>=tm-tpk & nk*vk_1<tM-tpk
                        alpah_k=(tm-tpk-nk*vk_1)/(nk*nk_1_vertical');
                        bk_tmp=0;
                    else
                        bk_tmp=0;
                    end
%                     if nk*vk_1>=tm-tpk & nk*vk_1<tM-tpk
%                         alpah_k=(tm-tpk-nk*vk_1)/(nk*nk_1_vertical');
%                         bk_tmp=0;
%                     end
                end
                if (alpah_k<alpah_v) & alpah_k>=1e-6
                    alpah_v=alpah_k;
                    l=k;
                    find2=1;
                    nk_1_vertical_final=nk_1_vertical;
                    bk=bk_tmp;
                else
                    
                end
            end
        else
            find2=0;
        end
    end
    if find2==0 || count>1000
        t=[0 0 0 0 0 0 0 0]';
        bool=0;
%         disp("索力分布无解");
        break
    else
        vk=vk_1+alpah_v.*nk_1_vertical_final';
        nk=N(l,:);
        langda_select=[langda_select,vk];
    %     line_select(1,:)=line_select(2,:);
    %     line_select(2,:)=l;
        line_select(1)=l;
        lk=l;
        k_vector=setdiff(k_vector_all,line_select);
        vk_2=vk_1;
        vk_1=vk;
        nk_2=nk_1;
        nk_1=nk;
        bk_2=bk_1;
        bk_1=bk;
        lk_2=lk_1;
        lk_1=lk;
    %     alpah_v=[1e10;1e10];
        alpah_v=[1e30];

        if ~ismember(l,line_find)
            line_find=[line_find;l];
            line_find=sort(line_find);
            vf=vk;
            vf_count=count+1;
        else
            if abs(vf(1)-vk(1))<1e-3 & abs(vf(2)-vk(2))<1e-3
                line_find=sort(line_find);
                if isequal(line_find,k_vector_all)
%                     disp('查找成功');
                    bool=1;
                    break;
                else
                    t=[0 0 0 0 0 0 0 0]';
                    bool=0;
%                     disp('查找失败');
                    return
                end
            else
                line_find=line_find;
            end
        end        
    end
    
end

langda_final_vce=langda_select(1:2,end-(size(langda_select,2)-vf_count):end-1);

%% 重心法得到多边形质心
% 求解A
A=0;
vc1=0;
vc2=0;

count=size(langda_select,2)-vf_count;

if count==3
    vc1=(langda_final_vce(1,1)+langda_final_vce(1,2)+langda_final_vce(1,3))/3;
    vc2=(langda_final_vce(2,1)+langda_final_vce(2,2)+langda_final_vce(2,3))/3;
end

if count==4
    vc1=(langda_final_vce(1,1)+langda_final_vce(1,2)+langda_final_vce(1,3)+langda_final_vce(1,4))/4;
    vc2=(langda_final_vce(2,1)+langda_final_vce(2,2)+langda_final_vce(2,3)+langda_final_vce(2,4))/4;
end

if count>4
    for p=1:size(langda_final_vce,2)-1
        A=A+(langda_final_vce(1,p)*langda_final_vce(2,p+1)-langda_final_vce(1,p+1)*langda_final_vce(2,p))/2;
    end

    for p=1:size(langda_final_vce,2)-1
        vc1=vc1+((langda_final_vce(1,p)+langda_final_vce(1,p+1))*(langda_final_vce(1,p)*langda_final_vce(2,p+1)-langda_final_vce(1,p+1)*langda_final_vce(2,p)))/(6*A);
        vc2=vc2+((langda_final_vce(2,p)+langda_final_vce(2,p+1))*(langda_final_vce(1,p)*langda_final_vce(2,p+1)-langda_final_vce(1,p+1)*langda_final_vce(2,p)))/(6*A);
    end
end

% vc1=456.6389;
% vc2=534.3178;

t=zeros(8,1);

langda_final=[vc1 vc2]';
t=tp+N*langda_final;

end

== matlab function Control_Scheme_Cartesian_PID_Simulink/MATLAB Function ==
  data: p input; f output; p_dot input; p_ddot input; theta input; theta_dot input; theta_ddot input
function f  = Inverse_Dynamics_Func(p,p_dot,p_ddot,theta,theta_dot,theta_ddot)
% CDPRs的动力学求解
% 输入:p,p_dot,p_ddot,theta,theta_dot,theta_ddot 位置与姿态及其各阶导数
% 输出:f 动平台产生的wrench
mp=79;          %动平台质量
g=9.81;
cp=[0 -0.075 0]'; %动平台COM相对于动平台的原点的位置偏移
IG=[1 0 0;0 1 0;0 0 1]; %动平台相对于动平台坐标系的惯性矩阵

% x_dot=[p_dot;theta_dot];
% x_ddot=[p_ddot;theta_ddot];
x_dot=[p_dot;theta_dot];
x_ddot=[p_ddot;theta_ddot];

%% 得到旋转矩阵
Rxyz=Theta2RotationMatrix_Func(theta(1),theta(2),theta(3));

%% 得到S(x),在得到平台在世界坐标系下的角速度omiga,进而得到omiga^是omiga对应的斜对称矩阵
thetax=theta(1);
thetay=theta(2);
thetaz=theta(3);

thetax_dot=theta_dot(1);
thetay_dot=theta_dot(2);
thetaz_dot=theta_dot(3);

Sx=[1 0 sind(thetay); 0 cosd(thetax) -sind(thetax)*cosd(thetay); 0 sind(thetax) cosd(thetax)*cosd(thetay)];
omiga=Sx*theta_dot;
v1=omiga(1);
v2=omiga(2);
v3=omiga(3);
omiga_sharp=[0 -v3 v2;v3 0 -v1;-v2 v1 0];
Sx=[eye(3,3) zeros(3,3); zeros(3,3) Sx];

%% 得到S_dot_(x,x_dot)的每个元素为S(x)相应位置元素的导数
Sx_dot_2_2=[0 0 cosd(thetay)*thetay_dot;0 -sind(thetax)*thetax_dot -cosd(thetax)*cosd(thetay)*thetax_dot+sind(thetax)*sind(thetay)*thetay_dot; 0 cosd(thetax)*thetax_dot -sind(thetax)*cosd(thetay)*thetax_dot-cosd(thetax)*sind(thetay)*thetay_dot];
Sx_dot=[zeros(3,3) zeros(3,3);zeros(3,3) Sx_dot_2_2];
% Sx_dot=zeros(6,6); %简化使得导数均为0

%% 通过cp得到c(x)=Rxyz*cp,进而得到c^(x)是c(x)对应的斜对称矩阵
cx=Rxyz*cp;
v1=cx(1);
v2=cx(2);
v3=cx(3);
c_sharp_x=[0 -v3 v2;v3 0 -v1;-v2 v1 0];

%% 得到g(x)
gx=mp*g*[0 0 -1 -cx(2) cx(1) 0]';

%% 得到H(x)=Rxyz*IG*Rxyz'+mp*c_sharp_x*c_sharp_x';
Hx=Rxyz*IG*Rxyz'+mp*c_sharp_x*c_sharp_x';

%% 得到M'(x)
M_apo_x=[mp*ones(3,3) -mp*c_sharp_x; mp*c_sharp_x Hx];

%% 得到C'(x)
C_apo_x=[mp*omiga_sharp*omiga_sharp*cx; omiga_sharp*Hx*omiga];

%% 最终得到动平台上wrench f
f=(M_apo_x*(Sx_dot*x_dot+Sx*x_ddot)+C_apo_x-gx);
end

== matlab function Control_Scheme_Cartesian_PID_Simulink/MATLAB Function2 ==
  data: p_dot input; theta_dot input; l_dot output; p input; theta input; q_dot output
function [l_dot,q_dot] = Jacobian_Func(p_dot,theta_dot,p,theta)
% 雅可比矩阵，从位姿x到绳长l，再到电机角度q

x=theta(1);
y=theta(2);
z=theta(3);
Rxyz=Theta2RotationMatrix_Func(x,y,z);

%% CoGiRo的参数 8绳索6自由度的CDPRs
% ai的定义
a1=[-7.5 -5.5 6]';
a2=[-7.5 -5.5 6]';
a3=[-7.5 5.5 6]';
a4=[-7.5 5.5 6]';
a5=[7.5 5.5 6]';
a6=[7.5 5.5 6]';
a7=[7.5 -5.5 6]';
a8=[7.5 -5.5 6]';
% bi的定义
b1=Rxyz*[0.5 -0.5 0]';
b2=Rxyz*[-0.5 0.5 1]';
b3=Rxyz*[-0.5 -0.5 0]';
b4=Rxyz*[0.5 0.5 1]';
b5=Rxyz*[-0.5 0.5 0]';
b6=Rxyz*[0.5 -0.5 1]';
b7=Rxyz*[0.5 0.5 0]';
b8=Rxyz*[-0.5 -0.5 1]';
% 绳索张力的上下限
tM=1000;
tm=10;
%% li=ai-bi-p,然后归一化li得到si=li/norm(li)
% li=ai-bi-p
l1=a1-b1-p;
l2=a2-b2-p;
l3=a3-b3-p;
l4=a4-b4-p;
l5=a5-b5-p;
l6=a6-b6-p;
l7=a7-b7-p;
l8=a8-b8-p;
% for i=1:8
%     expr=['l',num2str(i),'=a',num2str(i),'-b',num2str(i),'-p;'];
%     eval(expr);
% end
% si=li/norm(li)
s1=l1/norm(l1);
s2=l2/norm(l2);
s3=l3/norm(l3);
s4=l4/norm(l4);
s5=l5/norm(l5);
s6=l6/norm(l6);
s7=l7/norm(l7);
s8=l8/norm(l8);
% for i=1:8
%     expr=['s',num2str(i),'=l',num2str(i),'./norm(l',num2str(i),');'];
%     eval(expr);
% end

%% 构建W矩阵
% wi=[si;cross(bi,si)]
w1=[s1;cross(b1,s1)];
w2=[s2;cross(b2,s2)];
w3=[s3;cross(b3,s3)];
w4=[s4;cross(b4,s4)];
w5=[s5;cross(b5,s5)];
w6=[s6;cross(b6,s6)];
w7=[s7;cross(b7,s7)];
w8=[s8;cross(b8,s8)];
W=[w1 w2 w3 w4 w5 w6 w7 w8];

%% 得到雅可比矩阵
J=-W';

x_dot=[p_dot;theta_dot];

l_dot=J*x_dot;
q_dot=l_dot/0.0225;

end

== matlab function Control_Scheme_Cartesian_PID_Simulink/MATLAB Function3 ==
  data: q_dot input; p_dot output; p input; theta input; theta_dot output
function [p_dot,theta_dot] = Inverse_Jacobian_Func(q_dot,p,theta)
% 雅可比矩阵，从位姿x到绳长l，再到电机角度q

x=theta(1);
y=theta(2);
z=theta(3);
Rxyz=Theta2RotationMatrix_Func(x,y,z);

%% CoGiRo的参数 8绳索6自由度的CDPRs
% ai的定义
a1=[-7.5 -5.5 6]';
a2=[-7.5 -5.5 6]';
a3=[-7.5 5.5 6]';
a4=[-7.5 5.5 6]';
a5=[7.5 5.5 6]';
a6=[7.5 5.5 6]';
a7=[7.5 -5.5 6]';
a8=[7.5 -5.5 6]';
% bi的定义
b1=Rxyz*[0.5 -0.5 0]';
b2=Rxyz*[-0.5 0.5 1]';
b3=Rxyz*[-0.5 -0.5 0]';
b4=Rxyz*[0.5 0.5 1]';
b5=Rxyz*[-0.5 0.5 0]';
b6=Rxyz*[0.5 -0.5 1]';
b7=Rxyz*[0.5 0.5 0]';
b8=Rxyz*[-0.5 -0.5 1]';
% 绳索张力的上下限
tM=1000;
tm=10;
%% li=ai-bi-p,然后归一化li得到si=li/norm(li)
% li=ai-bi-p
l1=a1-b1-p;
l2=a2-b2-p;
l3=a3-b3-p;
l4=a4-b4-p;
l5=a5-b5-p;
l6=a6-b6-p;
l7=a7-b7-p;
l8=a8-b8-p;
% for i=1:8
%     expr=['l',num2str(i),'=a',num2str(i),'-b',num2str(i),'-p;'];
%     eval(expr);
% end
% si=li/norm(li)
s1=l1/norm(l1);
s2=l2/norm(l2);
s3=l3/norm(l3);
s4=l4/norm(l4);
s5=l5/norm(l5);
s6=l6/norm(l6);
s7=l7/norm(l7);
s8=l8/norm(l8);
% for i=1:8
%     expr=['s',num2str(i),'=l',num2str(i),'./norm(l',num2str(i),');'];
%     eval(expr);
% end

%% 构建W矩阵
% wi=[si;cross(bi,si)]
w1=[s1;cross(b1,s1)];
w2=[s2;cross(b2,s2)];
w3=[s3;cross(b3,s3)];
w4=[s4;cross(b4,s4)];
w5=[s5;cross(b5,s5)];
w6=[s6;cross(b6,s6)];
w7=[s7;cross(b7,s7)];
w8=[s8;cross(b8,s8)];
W=[w1 w2 w3 w4 w5 w6 w7 w8];

%% 得到雅可比矩阵
J=-W';
J_plus=pinv(J);
l_dot=q_dot*0.0225;
x_dot=J_plus*l_dot;
p_dot=x_dot(1:3,:);
theta_dot=x_dot(4:6,:);
% if theta_dot(1)<1e-3
%     theta_dot(1)=0;
% end
% if theta_dot(2)<1e-3
%     theta_dot(2)=0;
% end
% if theta_dot(3)<1e-3
%     theta_dot(3)=0;
% end
end

== matlab function Control_Scheme_Cartesian_PID_Simulink/MATLAB Function4 ==
  data: p input; l_len output; theta input; q output
function [l_len,q]  = InverseKenematics_Func(p,theta)
%UNTITLED3 求解CDPRs的逆运动学解
%   Detailed explanation goes here
x=theta(1);
y=theta(2);
z=theta(3);
Rxyz=Theta2RotationMatrix_Func(x,y,z);
%% CoGiRo的参数 8绳索6自由度的CDPRs
% ai的定义
a1=[-7.5 -5.5 6]';
a2=[-7.5 -5.5 6]';
a3=[-7.5 5.5 6]';
a4=[-7.5 5.5 6]';
a5=[7.5 5.5 6]';
a6=[7.5 5.5 6]';
a7=[7.5 -5.5 6]';
a8=[7.5 -5.5 6]';
% bi的定义
b1=[0.5 -0.5 0]';
b2=[-0.5 0.5 1]';
b3=[-0.5 -0.5 0]';
b4=[0.5 0.5 1]';
b5=[-0.5 0.5 0]';
b6=[0.5 -0.5 1]';
b7=[0.5 0.5 0]';
b8=[-0.5 -0.5 1]';
%% 计算li=ai-xp-Rbi
l1=a1-p-Rxyz*b1;
l2=a2-p-Rxyz*b2;
l3=a3-p-Rxyz*b3;
l4=a4-p-Rxyz*b4;
l5=a5-p-Rxyz*b5;
l6=a6-p-Rxyz*b6;
l7=a7-p-Rxyz*b7;
l8=a8-p-Rxyz*b8;
% 求绳索向量的模长
l1_len=norm(l1);
l2_len=norm(l2);
l3_len=norm(l3);
l4_len=norm(l4);
l5_len=norm(l5);
l6_len=norm(l6);
l7_len=norm(l7);
l8_len=norm(l8);
% l=[l1 l2 l3 l4 l5 l6 l7 l8]';
l_len=[l1_len l2_len l3_len l4_len l5_len l6_len l7_len l8_len]';
q=l_len./0.0225;
end

== matlab function Control_Scheme_Cartesian_PID_Simulink/MATLAB Function5 ==
  data: tao_in input; q output; t_in input; q_1 input; q_dot_1 input; q_dot output
function [q,q_dot] = SCDPR_Func(tao_in,t_in,q_1,q_dot_1)
% 主要求解电机的动力学方程，通过给定电机转矩以及索力信息，得到电机的角度以及角速度
%   此处显示详细说明

% global tao;
tao=tao_in;
% global tt;
tt=t_in;
% global Im;
Im=[0.1 0.1 0.1 0.1 0.1 0.1 0.1 0.1 0.1]';
% global Fv;
Fv=[1 1 1 1 1 1 1 1]';
% global Fs;
Fs=[1 1 1 1 1 1 1 1]';
% global R;
R=[0.0225 0.0225 0.0225 0.0225 0.0225 0.0225 0.0225 0.0225]';

T=0.001;

q=zeros(8,1);
q_dot=zeros(8,1);


% 第1个微分方程
Y11=q_1(1);
Y21=q_dot_1(1);
% 解微分方程
[t,q1] = ode45(@vdp1,[0 T],[Y11; Y21],[],tao,tt,Im,Fv,Fs,R);
q(1)=q1(end,1);
q_dot(1)=q1(end,2);

% 第2个微分方程
Y12=q_1(2);
Y22=q_dot_1(2);
% 解微分方程
[t,q2] = ode45(@vdp2,[0 T],[Y12; Y22],[],tao,tt,Im,Fv,Fs,R);
q(2)=q2(end,1);
q_dot(2)=q2(end,2);

% 第3个微分方程
Y13=q_1(3);
Y23=q_dot_1(3);
% 解微分方程
[t,q3] = ode45(@vdp3,[0 T],[Y13; Y23],[],tao,tt,Im,Fv,Fs,R);
q(3)=q3(end,1);
q_dot(3)=q3(end,2);

% 第4个微分方程
Y14=q_1(4);
Y24=q_dot_1(4);
% 解微分方程
[t,q4] = ode45(@vdp4,[0 T],[Y14; Y24],[],tao,tt,Im,Fv,Fs,R);
q(4)=q4(end,1);
q_dot(4)=q4(end,2);

% 第5个微分方程
Y15=q_1(5);
Y25=q_dot_1(5);
% 解微分方程
[t,q5] = ode45(@vdp5,[0 T],[Y15; Y25],[],tao,tt,Im,Fv,Fs,R);
q(5)=q5(end,1);
q_dot(5)=q5(end,2);

% 第6个微分方程
Y16=q_1(6);
Y26=q_dot_1(6);
% 解微分方程
[t,q6] = ode45(@vdp6,[0 T],[Y16; Y26],[],tao,tt,Im,Fv,Fs,R);
q(6)=q6(end,1);
q_dot(6)=q6(end,2);

% 第7个微分方程
Y17=q_1(7);
Y27=q_dot_1(7);
% 解微分方程
[t,q7] = ode45(@vdp7,[0 T],[Y17; Y27],[],tao,tt,Im,Fv,Fs,R);
q(7)=q7(end,1);
q_dot(7)=q7(end,2);

% 第8个微分方程
Y18=q_1(8);
Y28=q_dot_1(8);
% 解微分方程
[t,q8] = ode45(@vdp8,[0 T],[Y18; Y28],[],tao,tt,Im,Fv,Fs,R);
q(8)=q8(end,1);
q_dot(8)=q8(end,2);

function dydt1 = vdp1(t,y,tao,tt,Im,Fv,Fs,R)
%     global tao;
%     global tt;
%     global Im;
%     global Fv;
%     global Fs;
%     global R;
    
    tao1=tao(1);
    tt1=tt(1);
    Im1=Im(1);
    Fv1=Fv(1);
    Fs1=Fs(1);
    R1=R(1);

    p = y(1);
    dp = y(2);
% 	ddp = -Im_inv*Fv*dp-Im_inv*Fs*sign(dp)+Im_inv*tao-Im_inv*R*tt;
    ddp = -Fv1/Im1*dp-Fs1/Im1*sign(dp)+tao1/Im1-R1/Im1*tt1;
    dydt1 = [dp; ddp];
end

function dydt2 = vdp2(t,y,tao,tt,Im,Fv,Fs,R)
%     global tao;
%     global tt;
%     global Im;
%     global Fv;
%     global Fs;
%     global R;
    
    tao2=tao(2);
    tt2=tt(2);
    Im2=Im(2);
    Fv2=Fv(2);
    Fs2=Fs(2);
    R2=R(2);

    p = y(1);
    dp = y(2);
% 	ddp = -Im_inv*Fv*dp-Im_inv*Fs*sign(dp)+Im_inv*tao-Im_inv*R*tt;
    ddp = -Fv2/Im2*dp-Fs2/Im2*sign(dp)+tao2/Im2-R2/Im2*tt2;
    dydt2 = [dp; ddp];
end

function dydt3 = vdp3(t,y,tao,tt,Im,Fv,Fs,R)
%     global tao;
%     global tt;
%     global Im;
%     global Fv;
%     global Fs;
%     global R;
    
    tao3=tao(3);
    tt3=tt(3);
    Im3=Im(3);
    Fv3=Fv(3);
    Fs3=Fs(3);
    R3=R(3);

    p = y(1);
    dp = y(2);
% 	ddp = -Im_inv*Fv*dp-Im_inv*Fs*sign(dp)+Im_inv*tao-Im_inv*R*tt;
    ddp = -Fv3/Im3*dp-Fs3/Im3*sign(dp)+tao3/Im3-R3/Im3*tt3;
    dydt3 = [dp; ddp];
end

function dydt4 = vdp4(t,y,tao,tt,Im,Fv,Fs,R)
%     global tao;
%     global tt;
%     global Im;
%     global Fv;
%     global Fs;
%     global R;
    
    tao4=tao(4);
    tt4=tt(4);
    Im4=Im(4);
    Fv4=Fv(4);
    Fs4=Fs(4);
    R4=R(4);

    p = y(1);
    dp = y(2);
% 	ddp = -Im_inv*Fv*dp-Im_inv*Fs*sign(dp)+Im_inv*tao-Im_inv*R*tt;
    ddp = -Fv4/Im4*dp-Fs4/Im4*sign(dp)+tao4/Im4-R4/Im4*tt4;
    dydt4 = [dp; ddp];
end

function dydt5 = vdp5(t,y,tao,tt,Im,Fv,Fs,R)
%     global tao;
%     global tt;
%     global Im;
%     global Fv;
%     global Fs;
%     global R;
    
    tao5=tao(5);
    tt5=tt(5);
    Im5=Im(5);
    Fv5=Fv(5);
    Fs5=Fs(5);
    R5=R(5);

    p = y(1);
    dp = y(2);
% 	ddp = -Im_inv*Fv*dp-Im_inv*Fs*sign(dp)+Im_inv*tao-Im_inv*R*tt;
    ddp = -Fv5/Im5*dp-Fs5/Im5*sign(dp)+tao5/Im5-R5/Im5*tt5;
    dydt5 = [dp; ddp];
end

function dydt6 = vdp6(t,y,tao,tt,Im,Fv,Fs,R)
%     global tao;
%     global tt;
%     global Im;
%     global Fv;
%     global Fs;
%     global R;
    
    tao6=tao(6);
    tt6=tt(6);
    Im6=Im(6);
    Fv6=Fv(6);
    Fs6=Fs(6);
    R6=R(6);

    p = y(1);
    dp = y(2);
% 	ddp = -Im_inv*Fv*dp-Im_inv*Fs*sign(dp)+Im_inv*tao-Im_inv*R*tt;
    ddp = -Fv6/Im6*dp-Fs6/Im6*sign(dp)+tao6/Im6-R6/Im6*tt6;
    dydt6 = [dp; ddp];
end


function dydt7 = vdp7(t,y,tao,tt,Im,Fv,Fs,R)
%     global tao;
%     global tt;
%     global Im;
%     global Fv;
%     global Fs;
%     global R;
    
    tao7=tao(7);
    tt7=tt(7);
    Im7=Im(7);
    Fv7=Fv(7);
    Fs7=Fs(7);
    R7=R(7);

    p = y(1);
    dp = y(2);
% 	ddp = -Im_inv*Fv*dp-Im_inv*Fs*sign(dp)+Im_inv*tao-Im_inv*R*tt;
    ddp = -Fv7/Im7*dp-Fs7/Im7*sign(dp)+tao7/Im7-R7/Im7*tt7;
    dydt7 = [dp; ddp];
end

function dydt8 = vdp8(t,y,tao,tt,Im,Fv,Fs,R)
%     global tao;
%     global tt;
%     global Im;
%     global Fv;
%     global Fs;
%     global R;
    
    tao8=tao(8);
    tt8=tt(8);
    Im8=Im(8);
    Fv8=Fv(8);
    Fs8=Fs(8);
    R8=R(8);

    p = y(1);
    dp = y(2);
% 	ddp = -Im_inv*Fv*dp-Im_inv*Fs*sign(dp)+Im_inv*tao-Im_inv*R*tt;
    ddp = -Fv8/Im8*dp-Fs8/Im8*sign(dp)+tao8/Im8-R8/Im8*tt8;
    dydt8 = [dp; ddp];
end
end

== matlab function Control_Scheme_Cartesian_PID_Simulink/MATLAB Function6 ==
  data: t input; q_1 output size=[8,1] [8..8]; qd input; qd_dot input; q input; q_dot input; q_dot_1 output
function [q_1,q_dot_1] = Select_q_and_q_dot(t,qd,qd_dot,q,q_dot)

q_1=zeros(8,1);
q_dot_1=zeros(8,1);

if t<=3e-3
    q_1=qd;
    q_dot_1=qd_dot;
else
    q_1=q;
    q_dot_1=q_dot;
%     q_dot_1=qd_dot;
end

end
